simulink model "sim_real_control_no_gyro"  (R2024b)
settings: Solver=VariableStepAuto  StartTime=0.0  StopTime=50.0  RelTol=1e-3
settings Model: Creator=romai  LastModifiedBy=romai

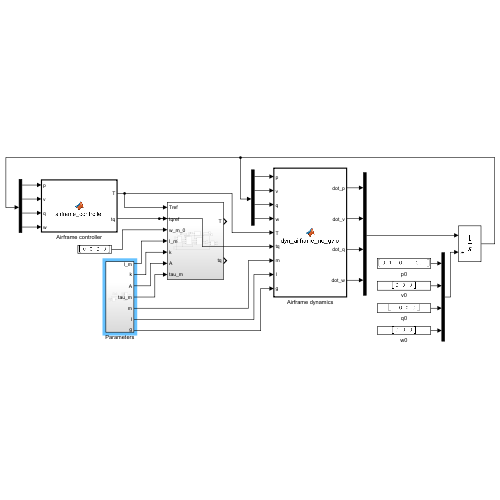
[thumbnail: Simulink's stored preview of the top-level diagram]
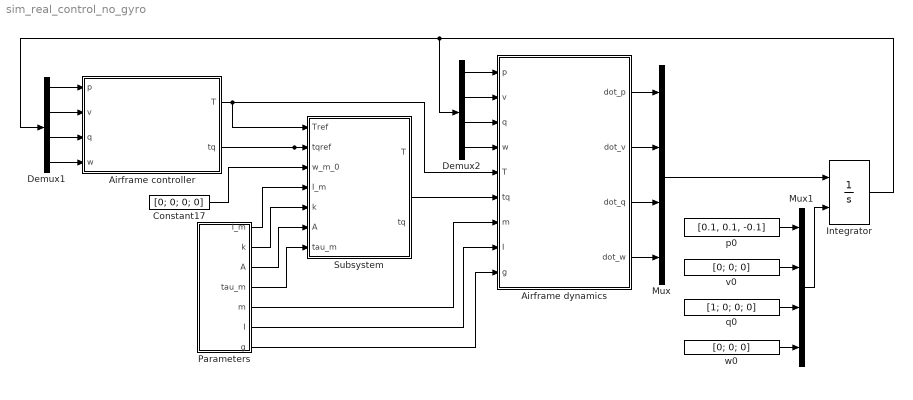
== system sim_real_control_no_gyro ==
  Airframe controller : MATLAB Function  TreatAsAtomicUnit=on
  Airframe dynamics : MATLAB Function  TreatAsAtomicUnit=on
  Constant17 : Constant  Value=[0; 0; 0; 0]
  Demux1 : Demux  Outputs=[3, 3, 4, 3]
  Demux2 : Demux  Outputs=[3, 3, 4, 3]
  Integrator : Integrator  InitialConditionSource=external
  Mux : Mux
  Mux1 : Mux
  Parameters : Subsystem
  Subsystem : Subsystem
  p0 : Constant  Value=[0.1, 0.1, -0.1]
  q0 : Constant  Value=[1; 0; 0; 0]
  v0 : Constant  Value=[0; 0; 0]
  w0 : Constant  Value=[0; 0; 0]
  wires:
  Mux1/1 -> Integrator/2
  Airframe dynamics/1(dot_p) -> Mux/1
  Demux2/2 -> Airframe dynamics/2(v)
  Mux/1 -> Integrator/1
  Airframe dynamics/4(dot_w) -> Mux/4
  Airframe dynamics/2(dot_v) -> Mux/2
  Integrator/1 -> Demux1/1, Demux2/1
  Airframe dynamics/3(dot_q) -> Mux/3
  Demux2/3 -> Airframe dynamics/3(q)
  Demux2/1 -> Airframe dynamics/1(p)
  Demux2/4 -> Airframe dynamics/4(w)
  Demux1/1 -> Airframe controller/1(p)
  Demux1/3 -> Airframe controller/3(q)
  Demux1/4 -> Airframe controller/4(w)
  v0/1 -> Mux1/2
  q0/1 -> Mux1/3
  p0/1 -> Mux1/1
  Demux1/2 -> Airframe controller/2(v)
  w0/1 -> Mux1/4
  Constant17/1 -> Subsystem/3(w_m_0)
  Airframe controller/1(T) -> Subsystem/1(Tref), Airframe dynamics/5(T)
  Airframe controller/2(tq) -> Subsystem/2(tqref), Airframe dynamics/6(tq)
  Parameters/1(I_m) -> Subsystem/4(I_m)
  Parameters/2(k) -> Subsystem/5(k)
  Parameters/3(A) -> Subsystem/6(A)
  Parameters/4(tau_m) -> Subsystem/7(tau_m)
  Parameters/5(m) -> Airframe dynamics/7(m)
  Parameters/6(I) -> Airframe dynamics/8(I)
  Parameters/7(g) -> Airframe dynamics/9(g)

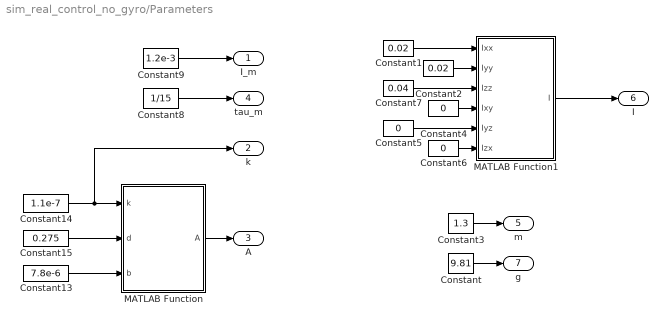
== system sim_real_control_no_gyro/Parameters ==
  Constant : Constant  Value=9.81
  Constant1 : Constant  Value=0.02
  Constant13 : Constant  Value=7.8e-6
  Constant14 : Constant  Value=1.1e-7
  Constant15 : Constant  Value=0.275
  Constant2 : Constant  Value=0.02
  Constant3 : Constant  Value=1.3
  Constant4 : Constant  Value=0
  Constant5 : Constant  Value=0
  Constant6 : Constant  Value=0
  Constant7 : Constant  Value=0.04
  Constant8 : Constant  Value=1/15
  Constant9 : Constant  Value=1.2e-3
  MATLAB Function : MATLAB Function  TreatAsAtomicUnit=on
  MATLAB Function1 : MATLAB Function  TreatAsAtomicUnit=on
  I_m : Outport
  k : Outport  Port=2
  A : Outport  Port=3
  tau_m : Outport  Port=4
  m : Outport  Port=5
  I : Outport  Port=6
  g : Outport  Port=7
  wires:
  Constant2/1 -> MATLAB Function1/2(Iyy)
  Constant5/1 -> MATLAB Function1/5(Iyz)
  Constant4/1 -> MATLAB Function1/4(Ixy)
  Constant7/1 -> MATLAB Function1/3(Izz)
  Constant1/1 -> MATLAB Function1/1(Ixx)
  Constant15/1 -> MATLAB Function/2(d)
  Constant6/1 -> MATLAB Function1/6(Izx)
  Constant13/1 -> MATLAB Function/3(b)
  MATLAB Function/1(A) -> A/1
  Constant8/1 -> tau_m/1
  Constant3/1 -> m/1
  Constant/1 -> g/1
  MATLAB Function1/1(I) -> I/1
  Constant9/1 -> I_m/1
  Constant14/1 -> MATLAB Function/1(k), k/1

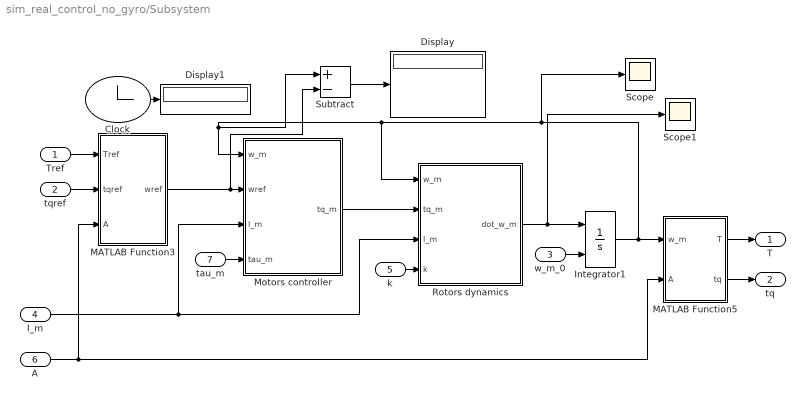
== system sim_real_control_no_gyro/Subsystem ==
  Tref : Inport
  tqref : Inport  Port=2
  w_m_0 : Inport  Port=3
  I_m : Inport  Port=4
  k : Inport  Port=5
  A : Inport  Port=6
  tau_m : Inport  Port=7
  Clock : Clock
  Display : Display
  Display1 : Display
  Integrator1 : Integrator  InitialConditionSource=external
  MATLAB Function3 : MATLAB Function  TreatAsAtomicUnit=on
  MATLAB Function5 : MATLAB Function  TreatAsAtomicUnit=on
  Motors controller : MATLAB Function  TreatAsAtomicUnit=on
  Rotors dynamics : MATLAB Function  TreatAsAtomicUnit=on
  Scope : Scope
  Scope1 : Scope
  Subtract : Sum  Inputs=+-
  T : Outport
  tq : Outport  Port=2
  wires:
  Rotors dynamics/1(dot_w_m) -> Scope1/1, Integrator1/1
  Motors controller/1(tq_m) -> Rotors dynamics/2(tq_m)
  MATLAB Function3/1(wref) -> Subtract/2, Motors controller/2(wref)
  tqref/1 -> MATLAB Function3/2(tqref)
  A/1 -> MATLAB Function5/2(A), MATLAB Function3/3(A)
  Integrator1/1 -> Scope/1, Rotors dynamics/1(w_m), Subtract/1, Motors controller/1(w_m), MATLAB Function5/1(w_m)
  Tref/1 -> MATLAB Function3/1(Tref)
  I_m/1 -> Rotors dynamics/3(I_m), Motors controller/3(I_m)
  tau_m/1 -> Motors controller/4(tau_m)
  MATLAB Function5/2(tq) -> tq/1
  MATLAB Function5/1(T) -> T/1
  w_m_0/1 -> Integrator1/2
  k/1 -> Rotors dynamics/4(k)
  Clock/1 -> Display1/1
  Subtract/1 -> Display/1

== matlab function sim_real_control_no_gyro/Subsystem/MATLAB Function5 ==
  data: w_m input; T output; tq output; A input
function [T, tq] = fcn(w_m, A)
    w_squared = w_m.^2;
    T = A(1,:) * w_squared;
    tq = A(2:4,:) * w_squared;
end

== matlab function sim_real_control_no_gyro/Airframe controller ==
  data: T output; tq output; p input; v input; q input; w input
function [T, tq] = airframe_controller(p,v,q,w)
    
    % Vertical component.
    %T = mg + 

    T = 15;
    tq = [0; 0; 0];
end

== matlab function sim_real_control_no_gyro/Airframe dynamics ==
  data: p input; dot_p output; v input; dot_v output; q input; w input; T input; tq input; m input; I input; g input; dot_q output; dot_w output
function [dot_p, dot_v, dot_q, dot_w] = dyn_airframe_no_gyro(p,v,q,w,T,tq,m,I,g)

    % Compute the time derivative of the state (p,v,q,w) of the drone's airframe, neglecting
    % the gyroscopic effects induced by the propellers.
    %
    % Inputs:
    %  - State variables:
    %   p       [3x1] Position.
    %   v       [3x1] Velocity.
    %   q       [4x1] Orientation to be interpreted as a unit quaternion (simulink doesn't support quaternion signals).
    %   w       [3x1] Angular velocity (in the drone's frame).
    %
    %  - Control variables:
    %   T       [1x1] Thrust generated by the 4 propellers.
    %   tq      [3x1] Torque generated by the 4 propellers (in the drone's frame).
    %
    %  - Constant parameters:
    %   m       [1x1] Mass of the drone.
    %   I       [3x3] Rotational inertia matrix of the drone (in the drone's frame).
    %   g       [1x1] Gravitational acceleration (positive).
    %
    % Outputs:
    %   dot_p   [3x1] Time derivative of position.
    %   dot_v   [3x1] Time derivative of velocity.
    %   dot_q   [4x1] Time derivative of orientation to be interpreted as a quaternion in T_q(S^3).
    %   dot_w   [3x1] Time derivative of angular velocity.
    
    q = quaternion(q');

    dot_p = v;
    dot_v = [0,0,-g] + T/m * rotatepoint(q, [0,0,1]);
    dot_q = compact(q * quaternion([0, w'/2]))'; % - (dot(q,q) - 1)^2;
    dot_w = I \ (tq - cross(w, I * w));
end

== matlab function sim_real_control_no_gyro/Parameters/MATLAB Function ==
  data: k input; d input; b input; A output
function A = fcn(k,d,b)
    
    db = d*b;

    A = [ b    b    b    b;
          0   db    0  -db;
         db    0  -db    0;
          k   -k    k   -k ];
end

== matlab function sim_real_control_no_gyro/Parameters/MATLAB Function1 ==
  data: Ixx input; I output; Iyy input; Izz input; Ixy input; Iyz input; Izx input
function I = fcn(Ixx, Iyy, Izz, Ixy, Iyz, Izx)
    
    I = [Ixx  Ixy  Izx;
         Ixy  Iyy  Iyz;
         Izx  Iyz  Izz];
end

== matlab function sim_real_control_no_gyro/Subsystem/MATLAB Function3 ==
  data: Tref input; wref output; tqref input; A input
function wref = fcn(Tref, tqref, A)
    w_squared = A \ [Tref; tqref];
    wref = sqrt(w_squared) .* [-1; 1; -1; 1];
end

== matlab function sim_real_control_no_gyro/Subsystem/Motors controller ==
  data: w_m input; wref input; tq_m output; I_m input; tau_m input
function tq_m = ESC(w_m, wref, I_m, tau_m)  % dot_wref ?
    tq_m = I_m * (-1/tau_m) * (w_m - wref);
end

== matlab function sim_real_control_no_gyro/Subsystem/Rotors dynamics ==
  data: w_m input; tq_m input; I_m input; dot_w_m output; k input
function dot_w_m  = dyn_rotors(w_m, tq_m, I_m, k)
    % Compute the time derivative of the angular velocities of the 4 rotors.
    %
    % Inputs:
    %   w_m    [4x1] Angular velocities of the 4 rotors.
    %   tq_m   [4x1] Torques generated by the 4 motors.
    %   I_m    [1x1] Single rotor (+ propeller?) rotational inertia with respect to its axis of rotation.
    %   k      [1x1] Drag parameter.
    %
    % Outputs:
    %   dot_w_m  [4x1] Time derivative of the angular velocities of the 4 rotors.

    drag = k * w_m .* abs(w_m);
    dot_w_m = (tq_m - drag) / I_m;
end
